simulink model "ID_lab_3_simulink"  (R2020b)
settings: Solver=VariableStepAuto  StartTime=0.0  StopTime=60  RelTol=1e-3
libraries: PoKeysIOInterface x1
settings Model: Creator=64190102  LastModifiedBy=64190102

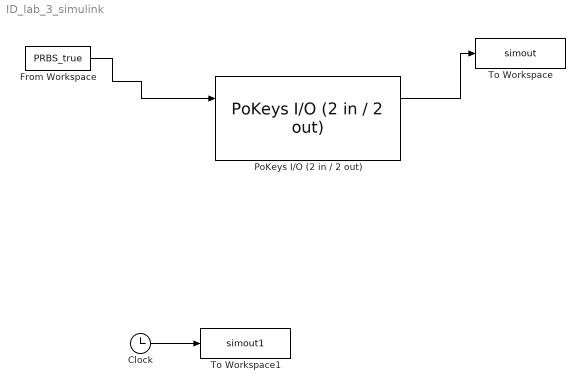
== system ID_lab_3_simulink ==
  Clock : Clock
  From Workspace : FromWorkspace  VariableName=PRBS_true  SampleTime=-1
  PoKeys I/O (2 in / 2 out) : PoKeysIOInterface/PoKeys I//O (2 in // 2 out)  MaxPowerLimit=100.0  IOTs=0.03  IOSerial=507
      settings: SourceProductName=PoKeys I/O interface
  To Workspace : ToWorkspace  VariableName=simout  SaveFormat=Timeseries  SampleTime=-1
  To Workspace1 : ToWorkspace  VariableName=simout1  SaveFormat=Timeseries  SampleTime=-1
  wires:
  From Workspace/1 -> PoKeys I/O (2 in / 2 out)/1
  PoKeys I/O (2 in / 2 out)/1 -> To Workspace/1
  Clock/1 -> To Workspace1/1
